simulink model "func6_a"  (R2016a)
settings: Solver=VariableStepAuto  StartTime=0.0  StopTime=10.0  RelTol=1e-3
libraries: basics_6_lib x1
settings Model: Creator=abehbood  LastModifiedBy=viswanad
settings GRTTargetCC: GeneratePreprocessorConditionals=Use local settings

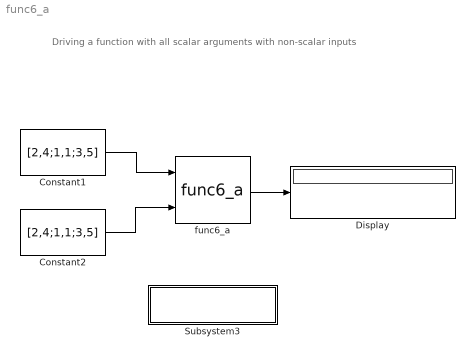
== system func6_a ==
  note: Driving a function with all scalar arguments with non-scalar inputs
  Constant1 : Constant  Value=[2,4;1,1;3,5]  OutDataTypeStr=int16  SampleTime=10
  Constant2 : Constant  Value=[2,4;1,1;3,5]  OutDataTypeStr=int16  SampleTime=10
  Display : Display
  Subsystem3 : Subsystem
      settings: OpenFcn=xmcOpenFileEx
      mask Display: disp(sprintf('Double Click to open\nthe main header file'))
  func6_a : basics_6_lib/func6_a  LibraryFunction=func6_a  IncludeFiles={'func6_a.h'}  SourceFiles={}  IncludeDirectories={}  TemplateParams={' '}  FunctionParamTypes={xmcDataType('void'); xmcDataType('int16_t'); xmcDataType('int16_t'); xmcDataType('int16_t &')}  FunctionParamPassbys={0.000000000000000000e+00; 0.000000000000000000e+00; 0.000000000000000000e+00; 1.000000000000000000e+00}  FunctionParamDimensions={'1'; '1'; '1'; '1'}  FunctionParamNames={'return'; 'in1'; 'in2'; 'out'}  FunctionParamDir={0.000000000000000000e+00; 1.000000000000000000e+00; 1.000000000000000000e+00; 2.000000000000000000e+00}  FunctionParamSupportsStreaming={false; false; false; false}  BufferDepth={'0'}  FunctionParamValues={'0'; '0'; '0'; '0'}
  wires:
  Constant1/1 -> func6_a/1
  Constant2/1 -> func6_a/2
  func6_a/1 -> Display/1

== system func6_a/Subsystem3 ==
